simulink model "TestSTARC_ABL_possible"  (R2017a)
settings: Solver=FixedStepDiscrete  StartTime=0.0  StopTime=10  FixedStep=0.015  RelTol=1e-3  EnableMultiTasking=on
libraries: Lib_PF_ActiveConvEffAC2DC_TMATS x2, Lib_PF_BusLoadDC_TMATS x2, Lib_Turbo_PGenerator_TMATS x2, Lib_PF_LineDC_TMATS x1, Lib_PF_BusLoadAC_TMATS x1, Lib_Solve_NormErr_TMATS x1, Lib_Solve_SSNRSolverJC_TMATS x1, Lib_PF_BusSlackAC_TMATS x1
settings Model: Creator=jwchapm2  LastModifiedBy=glthoma1
settings DataIOCC: LimitDataPoints=on  SaveFormat=Array
settings OptimizationCC: LifeSpan=inf
settings DebuggingCC: SFUnexpectedBacktrackingDiag=warning  SFNoUnconditionalDefaultTransitionDiag=warning  SFExecutionAtInitializationDiag=none
settings HardwareCC: ProdBitPerPointer=32  ProdBitPerSizeT=32  ProdBitPerPtrDiffT=32  ProdLargestAtomicFloat=None  ProdIntDivRoundTo=Undefined  ProdEndianess=Unspecified  ProdWordSize=32  ProdHWDeviceType=32-bit Generic
settings ModelReferenceCC: PropagateSignalLabelsOutOfModel=off
settings GRTTargetCC: TargetLangStandard=C89/C90 (ANSI)  GeneratePreprocessorConditionals=Disable all
settings ConfigComp: CovMetricSettings=dw  CovHtmlReporting=on  CovSaveCumulativeToWorkspaceVar=on  CovSaveSingleToWorkspaceVar=on  CovExternalEMLEnable=off

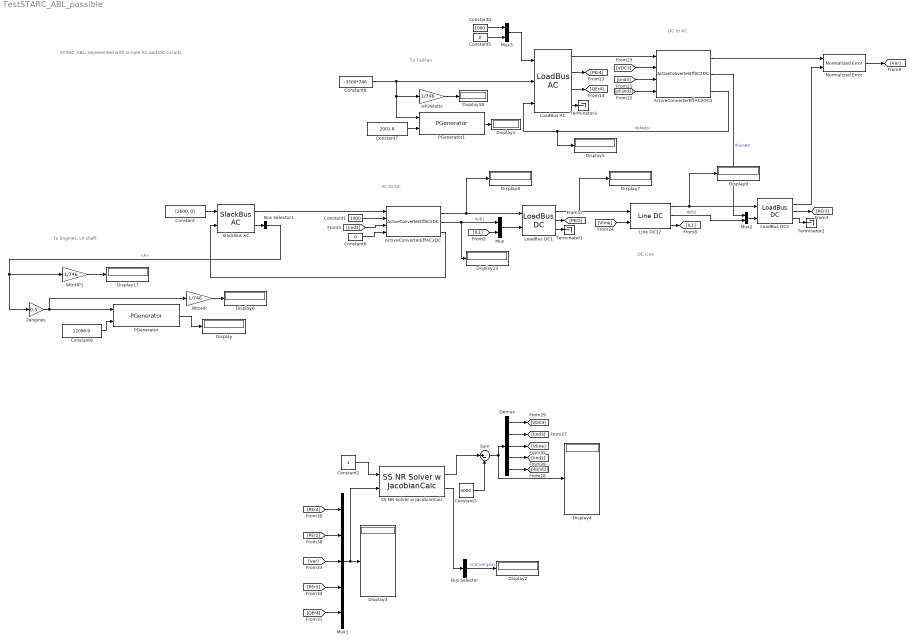
== system TestSTARC_ABL_possible ==
  note: To Engines, LP shaft
  note: AC to DC
  note: To TailFan
  note: DC Line
  note: DC to AC
  note: STARC_ABL,
      | represented with simple
      | AC and DC circuits
  2engines : Gain  Gain=0.5
  ActiveConverterEffAC2DC : Lib_PF_ActiveConvEffAC2DC_TMATS/ActiveConverterEffAC2DC  EffInEN_M=off  Eff_M=0.96  BlkNm_M=double(gcb)
  ActiveConverterEffAC2DC1 : Lib_PF_ActiveConvEffAC2DC_TMATS/ActiveConverterEffAC2DC  EffInEN_M=off  Eff_M=1/0.96  BlkNm_M=double(gcb)
  Bus Selector : BusSelector  OutputSignals=Converged
  Bus Selector1 : BusSelector  OutputSignals=P
  Constant : Constant  Value=[2000, 0]
  Constant1 : Constant  Value=1000
  Constant2 : Constant
  Constant3 : Constant  Value=5000
  Constant4 : Constant  Value=1000
  Constant5 : Constant  Value=0
  Constant6 : Constant  Value=0
  Constant7 : Constant  Value=2001.8
  Constant8 : Constant  Value=-3500*746
  Constant9 : Constant  Value=12096.9
  Demux : Demux  Outputs=5
  Display{,1..9,13,17..18} (13 alike) : Display
  HP2Watts : Gain  Gain=1/746
  Line DC12 : Lib_PF_LineDC_TMATS/Line DC  R_M=0.01
  LoadBus AC : Lib_PF_BusLoadAC_TMATS/LoadBus AC  PeInEN_M=on  P_M=-3500*746  QeInEN_M=off  Q_M=0  BlkNm_M=double(gcb)
  LoadBus DC1 : Lib_PF_BusLoadDC_TMATS/LoadBus DC  PeInEN_M=off  P_M=0  BlkNm_M=double(gcb)
  LoadBus DC2 : Lib_PF_BusLoadDC_TMATS/LoadBus DC  PeInEN_M=off  P_M=0  BlkNm_M=double(gcb)
  Mux : Mux  Inputs=2
  Mux1 : Mux  Inputs=5
  Mux2 : Mux  Inputs=2
  Mux3 : Mux  Inputs=2
  Normalized Error : Lib_Solve_NormErr_TMATS/Normalized Error
  PGenerator : Lib_Turbo_PGenerator_TMATS/PGenerator  Eff_M=1.01
  PGenerator1 : Lib_Turbo_PGenerator_TMATS/PGenerator  Eff_M=1.01
  SS NR Solver w JacobianCalc : Lib_Solve_SSNRSolverJC_TMATS/SS NR Solver w JacobianCalc  SJac_Per_M=[0.00001, 0.000001, 0.000001, 0.00001,0.000001]  SNR_IC_M="[1000  -2610  973    2710 0]+5000"  SNR_DX_M=5  SNR_Mx_M=100000  SNR_Mn_M=0.000001  SJacobianAttempts_M=20  Cond_Limits_M=1e-7
  SlackBus AC : Lib_PF_BusSlackAC_TMATS/SlackBus AC
  Sum : Sum  Inputs=|+-
  Terminator1 : Terminator
  Terminator2 : Terminator
  Terminator3 : Terminator
  WtoHP : Gain  Gain=1/746
  WtoHP1 : Gain  Gain=1/746
  wires:
  SlackBus AC/1 -> ActiveConverterEffAC2DC/1
  Constant/1 -> SlackBus AC/1
  ActiveConverterEffAC2DC/3 -> SlackBus AC/2
  ActiveConverterEffAC2DC/1 -> Display8/1, LoadBus DC1/1
  Constant1/1 -> ActiveConverterEffAC2DC/2
  Constant2/1 -> SS NR Solver w JacobianCalc/1
  [Iind1] -> ActiveConverterEffAC2DC/3
  Constant6/1 -> ActiveConverterEffAC2DC/4
  LoadBus DC1/2 -> [PEr2]
  SS NR Solver w JacobianCalc/1 -> Sum/1
  Mux1/1 -> SS NR Solver w JacobianCalc/2, Display3/1
  Sum/1 -> Display4/1, Demux/1
  Constant3/1 -> Sum/2
  SS NR Solver w JacobianCalc/2 -> Bus Selector/1
  Bus Selector/1 -> Display2/1  "<Converged>"
  LoadBus AC/1 -> ActiveConverterEffAC2DC1/1
  Line DC12/1 -> Display9/1, LoadBus DC2/1
  Mux/1 -> LoadBus DC1/2
  ActiveConverterEffAC2DC/2 -> Display13/1, Mux/1  "ItoB1"
  [IL1] -> Mux/2
  Line DC12/3 -> [IL1]
  ActiveConverterEffAC2DC1/2 -> Mux2/1  "IfromB2"
  Mux2/1 -> LoadBus DC2/2
  ActiveConverterEffAC2DC1/3 -> Display5/1, LoadBus AC/3  "ItoMotor"
  ActiveConverterEffAC2DC1/1 -> Normalized Error/1
  LoadBus DC2/1 -> Normalized Error/2
  LoadBus DC2/2 -> [PEr3]
  LoadBus AC/2 -> [PEr4]
  LoadBus AC/3 -> [QEr4]
  [Iind3] -> ActiveConverterEffAC2DC1/3
  [phiind3] -> ActiveConverterEffAC2DC1/4
  [VDC3] -> ActiveConverterEffAC2DC1/2
  [Vline] -> Line DC12/2
  Mux3/1 -> LoadBus AC/1
  Constant4/1 -> Mux3/1
  Demux/1 -> [VDC3]
  Demux/2 -> [Iind3]
  [Ver] -> Mux1/3
  [PEr3] -> Mux1/4
  [PEr4] -> Mux1/1
  [PEr2] -> Mux1/2
  Line DC12/2 -> Mux2/2  "ItoB2"
  Constant5/1 -> Mux3/2
  [QEr4] -> Mux1/5
  SlackBus AC/2 -> Bus Selector1/1
  Constant7/1 -> PGenerator1/2
  PGenerator/1 -> Display/1
  Bus Selector1/1 -> WtoHP1/1, 2engines/1  "<P>"
  Demux/3 -> [Vline]
  Demux/4 -> [Iind1]
  Demux/5 -> [phiind3]
  LoadBus DC2/3 -> Terminator2/1
  2engines/1 -> WtoHP/1, PGenerator/1
  LoadBus DC1/1 -> Display7/1, Line DC12/1
  Normalized Error/1 -> [Ver]
  WtoHP/1 -> Display6/1
  WtoHP1/1 -> Display17/1
  HP2Watts/1 -> Display18/1
  LoadBus DC1/3 -> Terminator1/1
  Constant8/1 -> PGenerator1/1, HP2Watts/1, LoadBus AC/2
  Constant9/1 -> PGenerator/2
  LoadBus AC/4 -> Terminator3/1
  PGenerator1/1 -> Display1/1
